simulink model "HW4_template_model"  (R2021a)
settings: Solver=VariableStepAuto  StartTime=0.0  StopTime=10.0  RelTol=1e-3
libraries: fl_lib x42, ee_lib x7, nesl_utility x6
settings Model: Creator=beave  LastModifiedBy=thana
settings SolverCC: AlgebraicLoopSolver=TrustRegion
settings DebuggingCC: SFMachineParentedDataDiag=warning

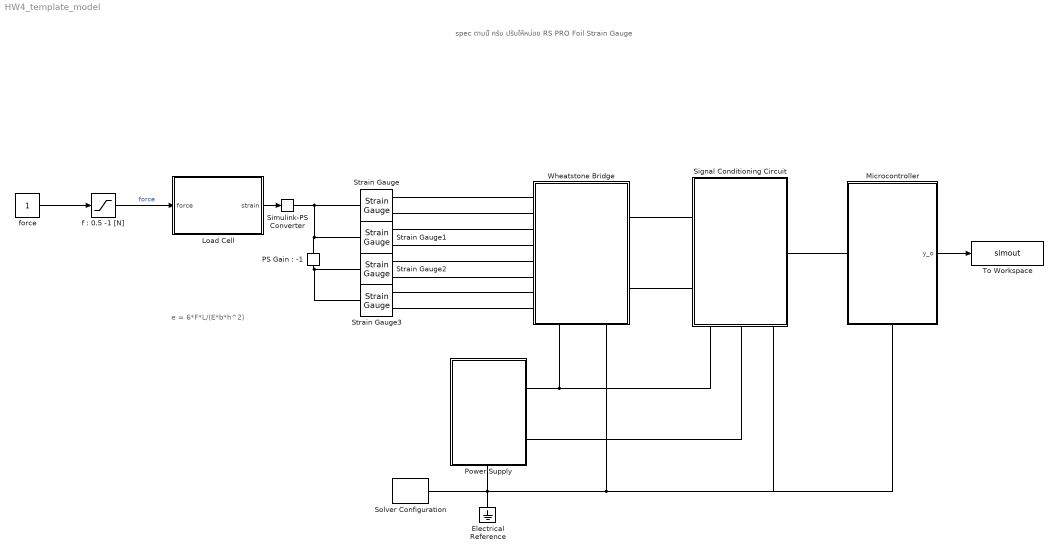
== system HW4_template_model ==
  note: e = 6*F*L/(E*b*h^2)
  note: spec ตามนี้ ครับ ปรับให้หน่อย RS PRO Foil Strain Gauge
  Electrical Reference : fl_lib/Electrical/Electrical Elements/Electrical Reference
  Load Cell : Subsystem
  Microcontroller : Subsystem
      settings: PortSchema="{\"entries\":[{\"content\":{\"sides\":[{\"content\":{\"connectorIds\":[\"LConn1\"]},\"type\":\"ConnectorPlacement.EquallySpacedRectSide\",\"uuid\":\"c8b31f12-36a9-42b7-b6a6-161bbb1c51b9\"},{\"content\":{\"connectorIds\":[\"Out1\"],\"side\":\"RIGHT\"},\"type\":\"ConnectorPlacement.EquallySpacedRectSide\",\"uuid\":\"adac1977-4ccc-4348-b89c-b647d4a007d6\"},{\"content\":{\"connectorIds\":[],\"side\":\"TOP\"},\"type\":\"ConnectorPlacement.EquallySpacedRectSide\",\"uuid\":\"3b0dd374-25f6-43e9-af40-0534b8c7b633\"},{\"content\":{\"connectorIds\":[\"RConn1\"],\"side\":\"BOTTOM\"},\"type\":\"ConnectorPlacement.EquallySpacedRectSide\",\"uuid\":\"a6b46765-0974-4448-9bf6-14b44e55447c\"},{\"content\":{\"connectorIds\":[],\"side\":\"HIDDEN\"},\"type\":\"ConnectorPlacement.EquallySpacedRectSide\",\"uuid\":\"1807c602-5a7a-4934-a0a9-e19cdde071ec\"}]},\"type\":\"ConnectorPlacement.EquallySpacedConnector\",\"uuid\":\"5e96f00e-4660-47d9-98e2-35dd8839db40\"}],\"packageUris\":[\"http://schema.mathworks.com/mf0/Connector/R2020b\"],\"version\":\"1.0\"}"
  "PS Gain : -1" : fl_lib/Physical Signals/Functions/PS Gain  gain=-1
  Power Supply : Subsystem
      settings: PortSchema="{\"entries\":[{\"content\":{\"sides\":[{\"content\":{\"connectorIds\":[]},\"type\":\"ConnectorPlacement.EquallySpacedRectSide\",\"uuid\":\"d484c286-8a66-4358-952e-0e35bb0e5568\"},{\"content\":{\"connectorIds\":[\"RConn1\",\"RConn2\"],\"side\":\"RIGHT\"},\"type\":\"ConnectorPlacement.EquallySpacedRectSide\",\"uuid\":\"128e18dd-1804-4321-ac62-61acca0b62f5\"},{\"content\":{\"connectorIds\":[],\"side\":\"TOP\"},\"type\":\"ConnectorPlacement.EquallySpacedRectSide\",\"uuid\":\"7b78cc83-63e5-401e-97d1-ae11342c6107\"},{\"content\":{\"connectorIds\":[\"RConn3\"],\"side\":\"BOTTOM\"},\"type\":\"ConnectorPlacement.EquallySpacedRectSide\",\"uuid\":\"16357e99-114e-457f-b57f-037bebe8facb\"},{\"content\":{\"connectorIds\":[],\"side\":\"HIDDEN\"},\"type\":\"ConnectorPlacement.EquallySpacedRectSide\",\"uuid\":\"e311646f-a995-48e7-a50f-2e5ca8d77595\"}]},\"type\":\"ConnectorPlacement.EquallySpacedConnector\",\"uuid\":\"3eb04d14-db36-4b49-95b1-e020a75bc06a\"}],\"packageUris\":[\"http://schema.mathworks.com/mf0/Connector/R2020b\"],\"version\":\"1.0\"}"
  Signal Conditioning Circuit : Subsystem
      settings: PortSchema="{\"entries\":[{\"content\":{\"sides\":[{\"content\":{\"connectorIds\":[\"LConn1\",\"LConn2\"]},\"type\":\"ConnectorPlacement.EquallySpacedRectSide\",\"uuid\":\"58874aca-5d10-42a9-8ce7-75e51f570882\"},{\"content\":{\"connectorIds\":[\"RConn1\"],\"side\":\"RIGHT\"},\"type\":\"ConnectorPlacement.EquallySpacedRectSide\",\"uuid\":\"2ca5ca46-eee6-4696-b8be-4fbc6f7a3b31\"},{\"content\":{\"connectorIds\":[],\"side\":\"TOP\"},\"type\":\"ConnectorPlacement.EquallySpacedRectSide\",\"uuid\":\"2ef733e7-6126-417c-8d34-0af4c6395645\"},{\"content\":{\"connectorIds\":[\"RConn2\",\"RConn3\",\"RConn4\"],\"side\":\"BOTTOM\"},\"type\":\"ConnectorPlacement.EquallySpacedRectSide\",\"uuid\":\"12614acf-d2ef-4b56-af04-15568bee15f7\"},{\"content\":{\"connectorIds\":[],\"side\":\"HIDDEN\"},\"type\":\"ConnectorPlacement.EquallySpacedRectSide\",\"uuid\":\"728fe90d-9968-4977-a19b-afe599b0e1ed\"}]},\"type\":\"ConnectorPlacement.EquallySpacedConnector\",\"uuid\":\"19f43891-d796-4a23-a4ed-658bd1b555a6\"}],\"packageUris\":[\"http://schema.mathworks.com/mf0/Connector/R2020b\"],\"version\":\"1.0\"}"
  Simulink-PS Converter : nesl_utility/Simulink-PS Converter  PhysicalDomain=network_engine_domain  SubClassName=ps_input  LeftPortType=input  RightPortType=output  PseudoPeriodic=off  Frequencies=[]  NoiseDistribution=none  NoiseParameters=[]  Unit=1  AffineConversion=off  FilteringAndDerivatives=provide  SimscapeFilterOrder=1  InputFilterTimeConstant=0.001  UdotUserProvided=0
      settings: SourceProductBaseCode=PW,SS
  Solver Configuration : nesl_utility/Solver Configuration  PhysicalDomain=network_engine_domain  SubClassName=solver  LeftPortType=input  RightPortType=generic  Tones=[]  Harmonics=[]  SimulateNoise=off  Profile=off  UseLocalSampling=off  EnableSwitchedLinearOptims=on  FrequencyDomain=off  UseCCode=off  RelTol=0.001  AbsTol=1e-06  MinStep=1e-09  ToWorkspace=off  RevertToSquareIcSolve=off  NumHomotopyIterations=100  PhasorMode=off  PhasorModeNumHarmonics=1  DoDC=off  ResidualTolerance=1e-09  UseLocalSolver=off  LocalSolverChoice=NE_BACKWARD_EULER_ADVANCER  LocalSolverSampleTime=0.001  DoFixedCost=off  MaxNonlinIter=3  MaxModeIter=2  ComputeImpulses=off  ImpulseIterations=2  LinearAlgebra=auto  EquationFormulation=NE_TIME_EF  DelaysMemoryBudget=1024  AutomaticFiltering=on  FilteringTimeConstant=0.001  PartitionStorageMethod=AS_NEEDED  PartitionMemoryBudget=1024  PartitionMethod=ROBUST
      settings: SourceProductBaseCode=PW,SS
  Strain Gauge{,1..3} (4 alike) : ee_lib/Sensors & Transducers/Strain Gauge  R=100 Ohm  K=2
      settings: SourceProductBaseCode=PS  InternalSimscapePortConfiguration="{\"Bottom\":[],\"Left\":[{\"id\":\"E\",\"label\":\"E\",\"type\":\"input\"}],\"Right\":[{\"id\":\"p\",\"label\":\"+\",\"type\":\"foundation.electrical.electrical\"},{\"id\":\"n\",\"label\":\"-\",\"type\":\"foundation.electrical.electrical\"}],\"Top\":[]}"
  To Workspace : ToWorkspace  VariableName=simout  SaveFormat=Timeseries  SampleTime=-1
  Wheatstone Bridge : Subsystem
      settings: PortSchema="{\"entries\":[{\"content\":{\"sides\":[{\"content\":{\"connectorIds\":[\"LConn1\",\"LConn2\",\"LConn3\",\"LConn4\",\"LConn5\",\"LConn6\",\"LConn7\",\"LConn8\"]},\"type\":\"ConnectorPlacement.EquallySpacedRectSide\",\"uuid\":\"a9dbb70d-760b-4500-9259-85d6974534e7\"},{\"content\":{\"connectorIds\":[\"RConn1\",\"RConn2\"],\"side\":\"RIGHT\"},\"type\":\"ConnectorPlacement.EquallySpacedRectSide\",\"uuid\":\"81dfe94d-60fd-4028-8d4c-e0668dffe582\"},{\"content\":{\"connectorIds\":[],\"side\":\"TOP\"},\"type\":\"ConnectorPlacement.EquallySpacedRectSide\",\"uuid\":\"2fdaeaef-2185-4af6-8e39-764e02e7f66d\"},{\"content\":{\"connectorIds\":[\"RConn3\",\"RConn4\"],\"side\":\"BOTTOM\"},\"type\":\"ConnectorPlacement.EquallySpacedRectSide\",\"uuid\":\"b11b3aa0-fdc3-4244-8b7b-b464348df7b0\"},{\"content\":{\"connectorIds\":[],\"side\":\"HIDDEN\"},\"type\":\"ConnectorPlacement.EquallySpacedRectSide\",\"uuid\":\"34f8aeea-abba-4e89-ba1e-4e54fe90c1fd\"}]},\"type\":\"ConnectorPlacement.EquallySpacedConnector\",\"uuid\":\"06e4c608-6193-4c2d-9c4d-84a3163f7e4d\"}],\"packageUris\":[\"http://schema.mathworks.com/mf0/Connector/R2020b\"],\"version\":\"1.0\"}"
  "f : 0.5 -1 [N]" : Saturate  UpperLimit=1  LowerLimit=0.5
  force : Constant
  wires:
  force/1 -> "f : 0.5 -1 [N]"/1
  Load Cell/1(strain) -> Simulink-PS Converter/1
  "f : 0.5 -1 [N]"/1 -> Load Cell/1(force)  "force"
  Microcontroller/1(y_o) -> To Workspace/1
  connections:
  Simulink-PS Converter/RConn1 -- Strain Gauge/LConn1 -- Strain Gauge1/LConn1 -- "PS Gain : -1"/LConn1
  Power Supply/RConn3 -- Microcontroller/RConn1 -- Signal Conditioning Circuit/RConn4 -- Wheatstone Bridge/RConn4 -- Solver Configuration/RConn1 -- Electrical Reference/LConn1
  Strain Gauge3/LConn1 -- Strain Gauge2/LConn1 -- "PS Gain : -1"/RConn1
  Power Supply/RConn1 -- Wheatstone Bridge/RConn3 -- Signal Conditioning Circuit/RConn2
  Power Supply/RConn2 -- Signal Conditioning Circuit/RConn3
  Strain Gauge/RConn1 -- Wheatstone Bridge/LConn1
  Strain Gauge/RConn2 -- Wheatstone Bridge/LConn2
  Strain Gauge1/RConn1 -- Wheatstone Bridge/LConn3
  Strain Gauge1/RConn2 -- Wheatstone Bridge/LConn4
  Strain Gauge2/RConn1 -- Wheatstone Bridge/LConn5
  Strain Gauge2/RConn2 -- Wheatstone Bridge/LConn6
  Strain Gauge3/RConn1 -- Wheatstone Bridge/LConn7
  Strain Gauge3/RConn2 -- Wheatstone Bridge/LConn8
  Signal Conditioning Circuit/RConn1 -- Microcontroller/LConn1
  Wheatstone Bridge/RConn1 -- Signal Conditioning Circuit/LConn1
  Wheatstone Bridge/RConn2 -- Signal Conditioning Circuit/LConn2

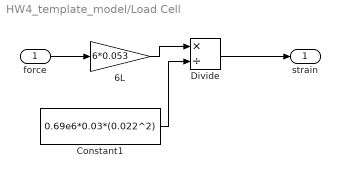
== system HW4_template_model/Load Cell ==
  force : Inport
  6L : Gain  Gain=6*0.053
  Constant1 : Constant  Value=0.69e6*0.03*(0.022^2)
  Divide : Product  Inputs=*/
  strain : Outport
  wires:
  force/1 -> 6L/1
  6L/1 -> Divide/1
  Constant1/1 -> Divide/2
  Divide/1 -> strain/1

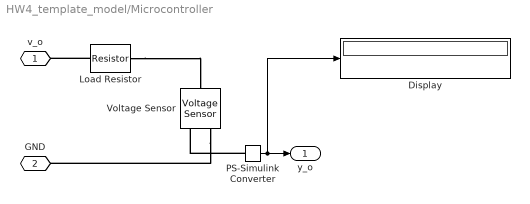
== system HW4_template_model/Microcontroller ==
  Display : Display
  "Load Resistor " : ee_lib/Passive/Resistor  R=1 Ohm  R_tol=5  enable_R_tol=0  tol_distribution=1  nSigma=4  enable_operating_limits=0  operating_limit_action=2  max_working_voltage=100 V  power_rating=1 W  enable_faults=0  fault_action=1  R_faulted=inf Ohm  enable_temporal_fault=0  t_fault=1 s  enable_behavioral_fault=0  max_permissible_current=1 A  t_fail_on_current=1 s  noise_mode=0  sample_time=1e-3 s  repeatability=1  auto_seed=3789891150  user_seed=0  Tdevice=25 degC  alpha=3.93e-3 1/K  Tmeas=25 degC  thermal_mass=100 J/K  power_derating_T1=70 degC  power_derating_T2=155 degC  operating_temperature_range_vec=[-50, 150] degC  temperature_specify=off  temperature_priority=High  temperature=298.15 K  temperature_nominal_specify=off  temperature_nominal_unit=K  temperature_nominal_value=1
  PS-Simulink Converter : nesl_utility/PS-Simulink Converter  PhysicalDomain=network_engine_domain  SubClassName=ps_output  LeftPortType=input  RightPortType=output  PseudoPeriodic=off  Frequencies=[]  Unit=inherit  AffineConversion=off
      settings: SourceProductBaseCode=PW,SS
  Voltage Sensor : fl_lib/Electrical/Electrical Sensors/Voltage Sensor
  v_o : PMIOPort  Side=Left
  GND : PMIOPort  Port=2  Side=Right
  y_o : Outport
  wires:
  PS-Simulink Converter/1 -> Display/1, y_o/1
  connections:
  "Load Resistor "/LConn1 -- v_o/RConn1
  "Load Resistor "/RConn1 -- Voltage Sensor/LConn1
  Voltage Sensor/RConn2 -- GND/RConn1
  PS-Simulink Converter/LConn1 -- Voltage Sensor/RConn1

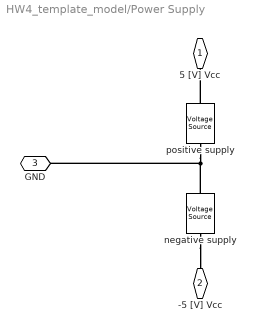
== system HW4_template_model/Power Supply ==
  negative supply : ee_lib/Sources/Voltage Source  dc_voltage=5 V  ac_voltage=0 V  ac_shift=0 rad  ac_frequency=60 Hz  noise_mode=0  PSD=0 V^2/Hz  repeatability=1  auto_seed=941108735  user_seed=0  sample_time=1e-3 s  i_specify=off  i_priority=None  i=0 A  i_nominal_specify=off  i_nominal_unit=A  i_nominal_value=1  v_specify=off  v_priority=None  v=0 V  v_nominal_specify=off  v_nominal_unit=V  v_nominal_value=1
  positive supply : ee_lib/Sources/Voltage Source  dc_voltage=5 V  ac_voltage=0 V  ac_shift=0 rad  ac_frequency=60 Hz  noise_mode=0  PSD=0 V^2/Hz  repeatability=1  auto_seed=223089112  user_seed=0  sample_time=1e-3 s  i_specify=off  i_priority=None  i=0 A  i_nominal_specify=off  i_nominal_unit=A  i_nominal_value=1  v_specify=off  v_priority=None  v=0 V  v_nominal_specify=off  v_nominal_unit=V  v_nominal_value=1
  5 [V] Vcc : PMIOPort  Side=Right
  -5 [V] Vcc : PMIOPort  Port=2  Side=Right
  GND : PMIOPort  Port=3  Side=Right
  connections:
  positive supply/RConn1 -- GND/RConn1 -- negative supply/LConn1
  positive supply/LConn1 -- 5 [V] Vcc/RConn1
  negative supply/RConn1 -- -5 [V] Vcc/RConn1

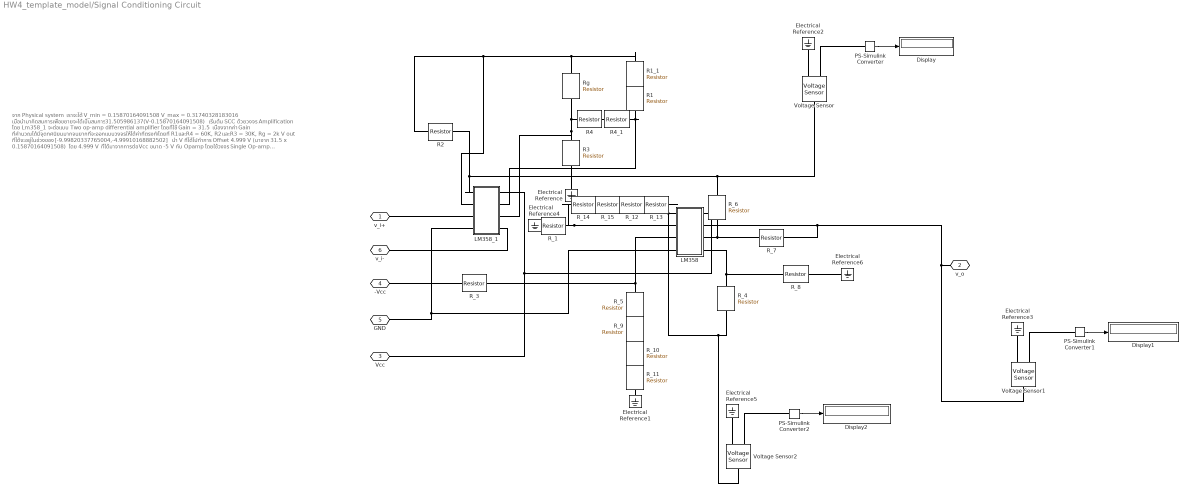
== system HW4_template_model/Signal Conditioning Circuit ==
  note: จาก Physical system เราจะได้
      | V_min = 0.15870164091508
      | V_max = 0.31740328183016
      |
      | เมื่อนำมาคิดสมการเพื่อขยายจะได้เป็นสมการ
      |
      | 31.505986137(V-0.15870164091508)
      |
      | เริ่มต้น SCC ด้วยวงจร Amplification โดย Lm358_1
      | จะต่อแบบ Two op-amp differential amplifier โดยที่ใช้ Gain = 31.5
      | เนื่องจากค่า Gain ที่คำนวณได้มีจุดทศนิยมมากจนยากที่จะออกแบบวงจรให้ได้ค่าที่ตรงกัน
      | โดยที่ R1และR4 = 60K, R2และR3 = 30K, Rg = 2k
      |
      | V out ที่ได้จะอยู่ในช่วงของ [-9.99820337765004,-4.99910168882502]
      |
      | นำ V ที่ได้ไปทำการ Offset 4.999 V (มาจาก 31.5 x 0.15870164091508)
      | โดย 4.999 V ที่ได้มาจากการต่อ Vcc ขนาด -5 V กับ Opamp
      | โดยใช้วงจร Single Op-amp differential amplifier โดยใช้ Gain = 0.9998
      | ทำให้ได้ v out ออกมา 4.999V
      |
      | นำ V out จาก Lm358_1 และ V out 4.999V เข้าวงจร Single Op-amp differential amplifier
      | โดยที่ 4.999 V ต่อเข้าขาบวก และ V out จาก Lm358_1 ต่อเข้าขาลบ โดยจะได้เป็นสมการ
      |
      | Vo = (-4.999 - (-Vout)) x Gain : gain = 1 เพื่อเป็นการ Offset เพียงอย่างเดียว
  Display : Display
  Display1 : Display
  Display2 : Display
  Electrical Reference{,1..6} (7 alike) : fl_lib/Electrical/Electrical Elements/Electrical Reference
  LM358 : Subsystem
  LM358_1 : Subsystem
  PS-Simulink Converter : nesl_utility/PS-Simulink Converter  PhysicalDomain=network_engine_domain  SubClassName=ps_output  LeftPortType=input  RightPortType=output  PseudoPeriodic=off  Frequencies=[]  Unit=inherit  AffineConversion=off
      settings: SourceProductBaseCode=PW,SS
  PS-Simulink Converter1 : nesl_utility/PS-Simulink Converter  PhysicalDomain=network_engine_domain  SubClassName=ps_output  LeftPortType=input  RightPortType=output  PseudoPeriodic=off  Frequencies=[]  Unit=inherit  AffineConversion=off
      settings: SourceProductBaseCode=PW,SS
  PS-Simulink Converter2 : nesl_utility/PS-Simulink Converter  PhysicalDomain=network_engine_domain  SubClassName=ps_output  LeftPortType=input  RightPortType=output  PseudoPeriodic=off  Frequencies=[]  Unit=inherit  AffineConversion=off
      settings: SourceProductBaseCode=PW,SS
  R{1..4} (4 alike) : fl_lib/Electrical/Electrical Elements/Resistor  R=30000 Ohm  i_specify=off  i_priority=None  i=0 A  i_nominal_specify=off  i_nominal_unit=A  i_nominal_value=1  v_specify=off  v_priority=None  v=0 V  v_nominal_specify=off  v_nominal_unit=V  v_nominal_value=1
  R1_1 : fl_lib/Electrical/Electrical Elements/Resistor  R=30000 Ohm  i_specify=off  i_priority=None  i=0 A  i_nominal_specify=off  i_nominal_unit=A  i_nominal_value=1  v_specify=off  v_priority=None  v=0 V  v_nominal_specify=off  v_nominal_unit=V  v_nominal_value=1
  R4_1 : fl_lib/Electrical/Electrical Elements/Resistor  R=30000 Ohm  i_specify=off  i_priority=None  i=0 A  i_nominal_specify=off  i_nominal_unit=A  i_nominal_value=1  v_specify=off  v_priority=None  v=0 V  v_nominal_specify=off  v_nominal_unit=V  v_nominal_value=1
  R_1 : fl_lib/Electrical/Electrical Elements/Resistor  R=10000 Ohm  i_specify=off  i_priority=None  i=0 A  i_nominal_specify=off  i_nominal_unit=A  i_nominal_value=1  v_specify=off  v_priority=None  v=0 V  v_nominal_specify=off  v_nominal_unit=V  v_nominal_value=1
  R_10 : fl_lib/Electrical/Electrical Elements/Resistor  R=68 Ohm  i_specify=off  i_priority=None  i=0 A  i_nominal_specify=off  i_nominal_unit=A  i_nominal_value=1  v_specify=off  v_priority=None  v=0 V  v_nominal_specify=off  v_nominal_unit=V  v_nominal_value=1
  R_11 : fl_lib/Electrical/Electrical Elements/Resistor  R=10 Ohm  i_specify=off  i_priority=None  i=0 A  i_nominal_specify=off  i_nominal_unit=A  i_nominal_value=1  v_specify=off  v_priority=None  v=0 V  v_nominal_specify=off  v_nominal_unit=V  v_nominal_value=1
  R_12 : fl_lib/Electrical/Electrical Elements/Resistor  R=68 Ohm  i_specify=off  i_priority=None  i=0 A  i_nominal_specify=off  i_nominal_unit=A  i_nominal_value=1  v_specify=off  v_priority=None  v=0 V  v_nominal_specify=off  v_nominal_unit=V  v_nominal_value=1
  R_13 : fl_lib/Electrical/Electrical Elements/Resistor  R=10 Ohm  i_specify=off  i_priority=None  i=0 A  i_nominal_specify=off  i_nominal_unit=A  i_nominal_value=1  v_specify=off  v_priority=None  v=0 V  v_nominal_specify=off  v_nominal_unit=V  v_nominal_value=1
  R_14 : fl_lib/Electrical/Electrical Elements/Resistor  R=9100 Ohm  i_specify=off  i_priority=None  i=0 A  i_nominal_specify=off  i_nominal_unit=A  i_nominal_value=1  v_specify=off  v_priority=None  v=0 V  v_nominal_specify=off  v_nominal_unit=V  v_nominal_value=1
  R_15 : fl_lib/Electrical/Electrical Elements/Resistor  R=820 Ohm  i_specify=off  i_priority=None  i=0 A  i_nominal_specify=off  i_nominal_unit=A  i_nominal_value=1  v_specify=off  v_priority=None  v=0 V  v_nominal_specify=off  v_nominal_unit=V  v_nominal_value=1
  R_3 : fl_lib/Electrical/Electrical Elements/Resistor  R=10000 Ohm  i_specify=off  i_priority=None  i=0 A  i_nominal_specify=off  i_nominal_unit=A  i_nominal_value=1  v_specify=off  v_priority=None  v=0 V  v_nominal_specify=off  v_nominal_unit=V  v_nominal_value=1
  R_{4,6..8} (4 alike) : fl_lib/Electrical/Electrical Elements/Resistor  R=1 Ohm  i_specify=off  i_priority=None  i=0 A  i_nominal_specify=off  i_nominal_unit=A  i_nominal_value=1  v_specify=off  v_priority=None  v=0 V  v_nominal_specify=off  v_nominal_unit=V  v_nominal_value=1
  R_5 : fl_lib/Electrical/Electrical Elements/Resistor  R=9100 Ohm  i_specify=off  i_priority=None  i=0 A  i_nominal_specify=off  i_nominal_unit=A  i_nominal_value=1  v_specify=off  v_priority=None  v=0 V  v_nominal_specify=off  v_nominal_unit=V  v_nominal_value=1
  R_9 : fl_lib/Electrical/Electrical Elements/Resistor  R=820 Ohm  i_specify=off  i_priority=None  i=0 A  i_nominal_specify=off  i_nominal_unit=A  i_nominal_value=1  v_specify=off  v_priority=None  v=0 V  v_nominal_specify=off  v_nominal_unit=V  v_nominal_value=1
  Rg : fl_lib/Electrical/Electrical Elements/Resistor  R=2000 Ohm  i_specify=off  i_priority=None  i=0 A  i_nominal_specify=off  i_nominal_unit=A  i_nominal_value=1  v_specify=off  v_priority=None  v=0 V  v_nominal_specify=off  v_nominal_unit=V  v_nominal_value=1
  Voltage Sensor : fl_lib/Electrical/Electrical Sensors/Voltage Sensor
  Voltage Sensor1 : fl_lib/Electrical/Electrical Sensors/Voltage Sensor
  Voltage Sensor2 : fl_lib/Electrical/Electrical Sensors/Voltage Sensor
  v_i+ : PMIOPort  Side=Left
  v_o : PMIOPort  Port=2  Side=Right
  Vcc : PMIOPort  Port=3  Side=Right
  -Vcc : PMIOPort  Port=4  Side=Right
  GND : PMIOPort  Port=5  Side=Right
  v_i- : PMIOPort  Port=6  Side=Left
  wires:
  PS-Simulink Converter/1 -> Display/1
  PS-Simulink Converter1/1 -> Display1/1
  PS-Simulink Converter2/1 -> Display2/1
  connections:
  Rg/RConn1 -- R2/LConn1 -- LM358_1/LConn2 -- R1_1/RConn1
  LM358/RConn3 -- R_7/LConn1 -- R_6/RConn1
  Vcc/RConn1 -- LM358/RConn1 -- LM358_1/RConn1
  LM358/RConn2 -- R_7/RConn1 -- Voltage Sensor1/LConn1 -- v_o/RConn1
  Rg/LConn1 -- LM358_1/RConn3 -- R3/RConn1 -- R4/LConn1
  R_3/RConn1 -- LM358/LConn3 -- R_5/LConn1
  R2/RConn1 -- LM358_1/LConn1 -- Voltage Sensor/LConn1 -- R_6/LConn1
  LM358_1/RConn2 -- R4_1/RConn1 -- R1/LConn1
  LM358/LConn4 -- GND/RConn1 -- LM358_1/LConn4
  v_i-/RConn1 -- LM358_1/RConn4
  v_i+/RConn1 -- LM358_1/LConn3
  R_10/RConn1 -- R_11/LConn1
  -Vcc/RConn1 -- R_3/LConn1
  Electrical Reference/LConn1 -- R3/LConn1
  R1/RConn1 -- R1_1/LConn1
  R4_1/LConn1 -- R4/RConn1
  Electrical Reference2/LConn1 -- Voltage Sensor/RConn2
  Voltage Sensor/RConn1 -- PS-Simulink Converter/LConn1
  Voltage Sensor1/RConn1 -- PS-Simulink Converter1/LConn1
  Electrical Reference3/LConn1 -- Voltage Sensor1/RConn2
  R_1/LConn1 -- Electrical Reference4/LConn1
  R_1/RConn1 -- R_14/LConn1 -- LM358/LConn2
  R_4/LConn1 -- Voltage Sensor2/LConn1 -- R_13/RConn1 -- LM358/LConn1
  Electrical Reference5/LConn1 -- Voltage Sensor2/RConn2
  Voltage Sensor2/RConn1 -- PS-Simulink Converter2/LConn1
  R_4/RConn1 -- R_8/LConn1 -- LM358/RConn4
  Electrical Reference6/LConn1 -- R_8/RConn1
  R_9/LConn1 -- R_5/RConn1
  Electrical Reference1/LConn1 -- R_11/RConn1
  R_10/LConn1 -- R_9/RConn1
  R_12/LConn1 -- R_15/RConn1
  R_12/RConn1 -- R_13/LConn1
  R_15/LConn1 -- R_14/RConn1

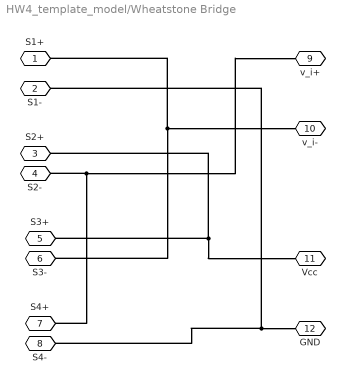
== system HW4_template_model/Wheatstone Bridge ==
  S1+ : PMIOPort  Side=Left
  S1- : PMIOPort  Port=2  Side=Left
  S2+ : PMIOPort  Port=3  Side=Left
  S2- : PMIOPort  Port=4  Side=Left
  S3+ : PMIOPort  Port=5  Side=Left
  S3- : PMIOPort  Port=6  Side=Left
  S4+ : PMIOPort  Port=7  Side=Left
  S4- : PMIOPort  Port=8  Side=Left
  v_i+ : PMIOPort  Port=9  Side=Right
  v_i- : PMIOPort  Port=10  Side=Right
  Vcc : PMIOPort  Port=11  Side=Right
  GND : PMIOPort  Port=12  Side=Right
  connections:
  S1-/RConn1 -- GND/RConn1 -- S4-/RConn1
  S2-/RConn1 -- v_i+/RConn1 -- S4+/RConn1
  S1+/RConn1 -- v_i-/RConn1 -- S3-/RConn1
  S2+/RConn1 -- Vcc/RConn1 -- S3+/RConn1

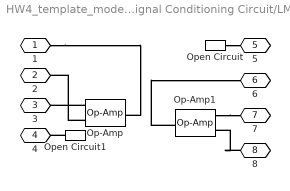
== system HW4_template_model/Signal Conditioning Circuit/LM358 ==
  Op-Amp : fl_lib/Electrical/Electrical Elements/Op-Amp  outI_specify=off  outI_priority=None  outI=0 A  outI_nominal_specify=off  outI_nominal_unit=A  outI_nominal_value=1
  Op-Amp1 : fl_lib/Electrical/Electrical Elements/Op-Amp  outI_specify=off  outI_priority=None  outI=0 A  outI_nominal_specify=off  outI_nominal_unit=A  outI_nominal_value=1
  Open Circuit : fl_lib/Electrical/Electrical Elements/Open Circuit  v_specify=off  v_priority=None  v=0 V  v_nominal_specify=off  v_nominal_unit=V  v_nominal_value=1
      settings: SourceProductBaseCode=SS
  Open Circuit1 : fl_lib/Electrical/Electrical Elements/Open Circuit  v_specify=off  v_priority=None  v=0 V  v_nominal_specify=off  v_nominal_unit=V  v_nominal_value=1
      settings: SourceProductBaseCode=SS
  1 : PMIOPort  Side=Left
  2 : PMIOPort  Port=2  Side=Left
  3 : PMIOPort  Port=3  Side=Left
  4 : PMIOPort  Port=4  Side=Left
  5 : PMIOPort  Port=5  Side=Right
  6 : PMIOPort  Port=6  Side=Right
  7 : PMIOPort  Port=7  Side=Right
  8 : PMIOPort  Port=8  Side=Right
  connections:
  Open Circuit/LConn1 -- 5/RConn1
  Open Circuit1/LConn1 -- 4/RConn1
  Op-Amp/LConn1 -- 3/RConn1
  Op-Amp/LConn2 -- 2/RConn1
  1/RConn1 -- Op-Amp/RConn1
  Op-Amp1/LConn2 -- 7/RConn1
  8/RConn1 -- Op-Amp1/LConn1
  Op-Amp1/RConn1 -- 6/RConn1

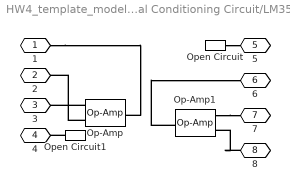
== system HW4_template_model/Signal Conditioning Circuit/LM358_1 ==
  Op-Amp : fl_lib/Electrical/Electrical Elements/Op-Amp  outI_specify=off  outI_priority=None  outI=0 A  outI_nominal_specify=off  outI_nominal_unit=A  outI_nominal_value=1
  Op-Amp1 : fl_lib/Electrical/Electrical Elements/Op-Amp  outI_specify=off  outI_priority=None  outI=0 A  outI_nominal_specify=off  outI_nominal_unit=A  outI_nominal_value=1
  Open Circuit : fl_lib/Electrical/Electrical Elements/Open Circuit  v_specify=off  v_priority=None  v=0 V  v_nominal_specify=off  v_nominal_unit=V  v_nominal_value=1
      settings: SourceProductBaseCode=SS
  Open Circuit1 : fl_lib/Electrical/Electrical Elements/Open Circuit  v_specify=off  v_priority=None  v=0 V  v_nominal_specify=off  v_nominal_unit=V  v_nominal_value=1
      settings: SourceProductBaseCode=SS
  1 : PMIOPort  Side=Left
  2 : PMIOPort  Port=2  Side=Left
  3 : PMIOPort  Port=3  Side=Left
  4 : PMIOPort  Port=4  Side=Left
  5 : PMIOPort  Port=5  Side=Right
  6 : PMIOPort  Port=6  Side=Right
  7 : PMIOPort  Port=7  Side=Right
  8 : PMIOPort  Port=8  Side=Right
  connections:
  Op-Amp1/RConn1 -- 6/RConn1
  8/RConn1 -- Op-Amp1/LConn1
  Op-Amp1/LConn2 -- 7/RConn1
  1/RConn1 -- Op-Amp/RConn1
  Op-Amp/LConn2 -- 2/RConn1
  Op-Amp/LConn1 -- 3/RConn1
  Open Circuit1/LConn1 -- 4/RConn1
  Open Circuit/LConn1 -- 5/RConn1
